simulink model "corBO"  (R2016b)
settings: Solver=VariableStepAuto  StartTime=0.0  StopTime=2  RelTol=1e-3
values from neighbouring files (symbols this model uses):
  f = 120    [Cons.m]
  Ki = 43.2/1000    (= 0.0432)    [Cons.m]
  Kred = 35.9    [Cons.m]
  meq = 120    [Cons.m]
  rpignon = 21*0.8/(2*1000)    (= 0.0084)    [Cons.m]
settings Model: Creator=canar  LastModifiedBy=emiliendurif

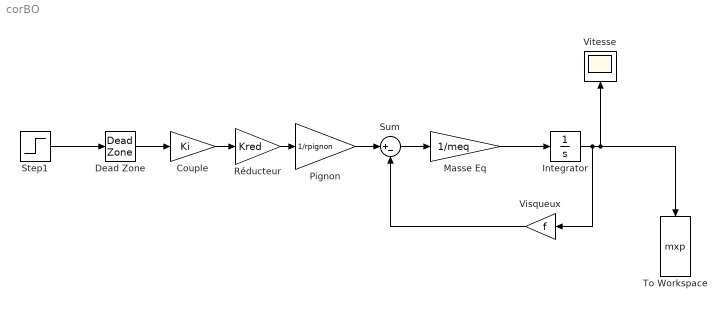
== system corBO ==
  Couple : Gain  Gain=Ki
  Dead Zone : DeadZone  LowerValue=-0.05  UpperValue=0.05  SaturateOnIntegerOverflow=on
  Integrator : Integrator
  Masse Eq : Gain  Gain=1/meq
  Pignon : Gain  Gain=1/rpignon
  Réducteur : Gain  Gain=Kred
  Step1 : Step  Time=0.1  After=0.2  SampleTime=0
  Sum : Sum  Inputs=|+-
  To Workspace : ToWorkspace  VariableName=mxp  SaveFormat=Timeseries  SampleTime=-1
  Visqueux : Gain  Gain=f
  Vitesse : Scope
  wires:
  Integrator/1 -> Visqueux/1, To Workspace/1, Vitesse/1
  Visqueux/1 -> Sum/2
  Réducteur/1 -> Pignon/1
  Step1/1 -> Dead Zone/1
  Couple/1 -> Réducteur/1
  Dead Zone/1 -> Couple/1
  Pignon/1 -> Sum/1
  Sum/1 -> Masse Eq/1
  Masse Eq/1 -> Integrator/1
